simulink model "dcmotor_closedloop_inner_twoloop"  (R2022b)
settings: Solver=ode5  StartTime=0.0  StopTime=3  MaxStep=10e-6  RelTol=1e-1  EnableMultiTasking=on
libraries: spsDiodeLib x6, spsCurrentMeasurementLib x3, spsVoltageMeasurementLib x3, spsSeriesRLCBranchLib x3, spsACVoltageSourceLib x3, powerlib_extras x2, spsMosfetLib x2, spspowerguiLib x1, spsDCMachineLib x1, spsDCVoltageSourceLib x1, spsNeutralLib x1
settings Model: Creator=g0305973  LastModifiedBy=e0927009
settings SolverCC: AlgebraicLoopSolver=TrustRegion
settings DataIOCC: LimitDataPoints=on  SaveFormat=Array  SignalLoggingSaveFormat=ModelDataLogs  ReturnWorkspaceOutputs=off  SignalLoggingName=sigsOut
settings OptimizationCC: ExpressionDepthLimit=2147483647  InitFltsAndDblsToZero=on  LifeSpan=inf
settings DebuggingCC: SaveWithParameterizedLinksMsg=none  UnderspecifiedInitializationDetection=Classic  MergeDetectMultiDrivingBlocksExec=none  SignalResolutionControl=TryResolveAllWithWarning  MultiTaskDSMMsg=warning  MultiTaskCondExecSysMsg=none  FcnCallInpInsideContextMsg=warning  UnconnectedInputMsg=warning  UnconnectedOutputMsg=warning  UnconnectedLineMsg=warning  StateNameClashWarn=warning  SFUnexpectedBacktrackingDiag=warning  SFNoUnconditionalDefaultTransitionDiag=warning  SFExecutionAtInitializationDiag=none  SFMachineParentedDataDiag=warning  ArithmeticOperatorsInVariantConditions=warning
settings HardwareCC: ProdBitPerPointer=32  ProdBitPerSizeT=32  ProdBitPerPtrDiffT=32  ProdLargestAtomicFloat=None  ProdIntDivRoundTo=Undefined  ProdEndianess=Unspecified  ProdWordSize=32  ProdHWDeviceType=32-bit Generic  TargetUnknown=on
settings ModelReferenceCC: EnableRefExpFcnMdlSchedulingChecks=on  PropagateSignalLabelsOutOfModel=off
settings SFSimCC: SimUseLocalCustomCode=off  CustomCodeUndefinedFunction=UseInterfaceOnly
settings RTWCC: RTWUseLocalCustomCode=off
settings CodeAppCC: StateflowObjectComments=on
settings GRTTargetCC: TargetFcnLib=ansi_tfl_tmw.mat  TargetLangStandard=C89/C90 (ANSI)  CombineOutputUpdateFcns=off  GRTInterface=on
settings ConfigComp: CovMetricSettings=dw  CovSaveCumulativeToWorkspaceVar=on  CovSaveSingleToWorkspaceVar=on  CovExternalEMLEnable=off
settings SimscapeCC: SimscapeNormalizeSystem=off

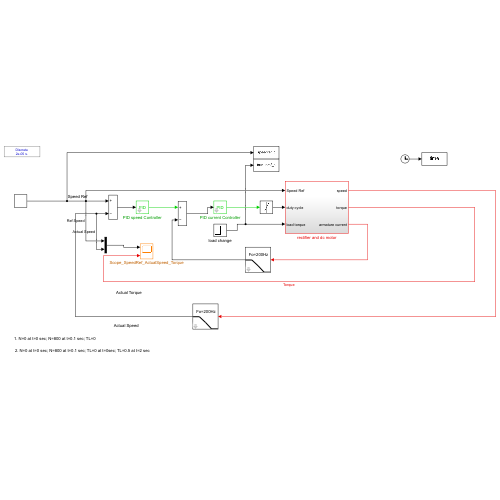
[thumbnail: Simulink's stored preview of the top-level diagram]
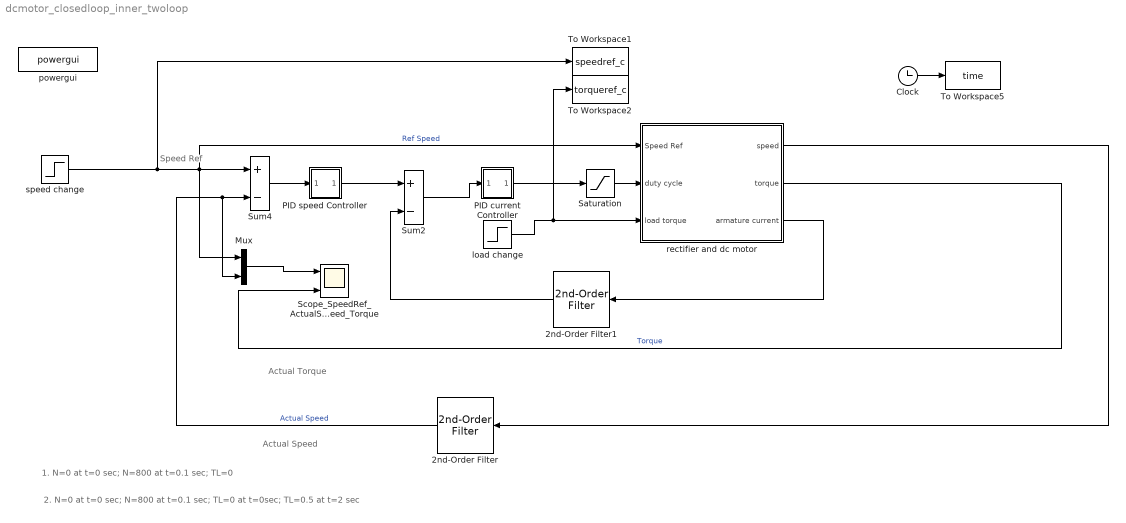
== system dcmotor_closedloop_inner_twoloop ==
  note: Speed Ref
  note: Actual Speed
  note: Actual Torque
  note: 2. N=0 at t=0 sec; N=800 at t=0.1 sec; TL=0 at t=0sec; TL=0.5 at t=2 sec
  note: 1. N=0 at t=0 sec; N=800 at t=0.1 sec; TL=0
  2nd-Order Filter : powerlib_extras/Control  Blocks/2nd-Order Filter  FilterType=Lowpass  Fo=200  Zeta=0.707  Initialize=off  Vac_Init=[1 45 60]  Vdc_Init=-0.5  PlotResponse=off  param1=[1 500 1]
  2nd-Order Filter1 : powerlib_extras/Control  Blocks/2nd-Order Filter  FilterType=Lowpass  Fo=200  Zeta=0.707  Initialize=off  Vac_Init=[1 45 60]  Vdc_Init=-0.5  PlotResponse=off  param1=[1 500 1]
  Clock : Clock
  Mux : Mux  Inputs=2
  PID current Controller : Subsystem  AncestorBlock=simulink_extras/Additional Linear/PID Controller  mask(PID Controller){P=0.4366, I=32.4627, D=0}
      mask prompts: P "Proportional:"; I "Integral:"; D "Derivative:"
      mask help:
      | Enter expressions for proportional, integral, and derivative terms.
      | P+I/s+Ds
      settings: LibrarySourceBlock=|
      | simulink_extras/Additional
      | Linear/PID Controller
      mask Help: This block implements a PID controller where parameters are entered for the Proportional, Integral and Derivative terms. Unmask this block to see how it works. The derivative term is implemented using a true derivative block.
      mask Display: disp('PID')
  PID speed Controller : Subsystem  AncestorBlock=simulink_extras/Additional Linear/PID Controller  mask(PID Controller){P=0.0256, I=0.0163, D=0}
      mask prompts: P "Proportional:"; I "Integral:"; D "Derivative:"
      mask help:
      | Enter expressions for proportional, integral, and derivative terms.
      | P+I/s+Ds
      settings: LibrarySourceBlock=|
      | simulink_extras/Additional
      | Linear/PID Controller
      mask Help: This block implements a PID controller where parameters are entered for the Proportional, Integral and Derivative terms. Unmask this block to see how it works. The derivative term is implemented using a true derivative block.
      mask Display: disp('PID')
  Saturation : Saturate  UpperLimit=1  LowerLimit=0
  Scope_SpeedRef_ActualSpeed_Torque : Scope  NumInputPorts=2
  Sum2 : Sum  Inputs=+-  SaturateOnIntegerOverflow=on
  Sum4 : Sum  Inputs=+-  SaturateOnIntegerOverflow=on
  To Workspace1 : ToWorkspace  VariableName=speedref_c  SampleTime=2e-5
  To Workspace2 : ToWorkspace  VariableName=torqueref_c  SampleTime=2e-5
  To Workspace5 : ToWorkspace  VariableName=time  SampleTime=2e-5
  load change : Step  Time=2  After=0.5  SampleTime=0
  powergui : spspowerguiLib/powergui  Priority=2  SimulationMode=Discrete  SampleTime=20e-6  frequency=60  Iterations=50  frequencyindice=50  Pbase=100e6  ErrMax=1e-4  UnitsV=kV  UnitsW=MW  buscounter=0  FunctionMessages=off  echomessages=off  EnableUseOfTLC=off  CurrentSourceSwitches=off  DisableSnubberDevices=off  DisableRonSwitches=off  DisableVfSwitches=off  DisplayEquations=off  AutomaticDiscreteSolvers=off  SolverType=Tustin  Interpol=off  ExternalGateDelay=off  methode=off  Ts=0  x0status=blocks  SPID=off  SwTol=0  HookPort=off  NonlinearTolerance=1e-4  nMaxIteration=100  ContinueOnMaxIteration=off  RestoreLinks=warning  ResistiveCurrentMeasurement=off  Frange=[0:2:500]  Ylog=off  Xlog=on  ShowGrid=off  save=off  variable=ZData  structure=0  ZoomFFT=on  StartTime=0.0  cycles=1  DisplayStyle=1  fundamental=60  FreqAxis=off  MaxFrequency=1000  frequencyindicesteady=1  RmsSteady=1  display=off
  rectifier and dc motor : Subsystem
  speed change : Step  Time=0.1  After=800  SampleTime=0
  wires:
  rectifier and dc motor/1(speed) -> 2nd-Order Filter/1
  Mux/1 -> Scope_SpeedRef_ActualSpeed_Torque/1
  Sum4/1 -> PID speed Controller/1(In_1)
  2nd-Order Filter/1 -> Sum4/2, Mux/2  "Actual Speed"
  speed change/1 -> Sum4/1, rectifier and dc motor/1(Speed Ref), Mux/1, To Workspace1/1  "Ref Speed"
  rectifier and dc motor/2(torque) -> Scope_SpeedRef_ActualSpeed_Torque/2  "Torque"
  load change/1 -> To Workspace2/1, rectifier and dc motor/3(load torque)
  Clock/1 -> To Workspace5/1
  Sum2/1 -> PID current Controller/1(In_1)
  rectifier and dc motor/3(armature current) -> 2nd-Order Filter1/1
  2nd-Order Filter1/1 -> Sum2/2
  PID current Controller/1(Out_1) -> Saturation/1
  PID speed Controller/1(Out_1) -> Sum2/1
  Saturation/1 -> rectifier and dc motor/2(duty cycle)

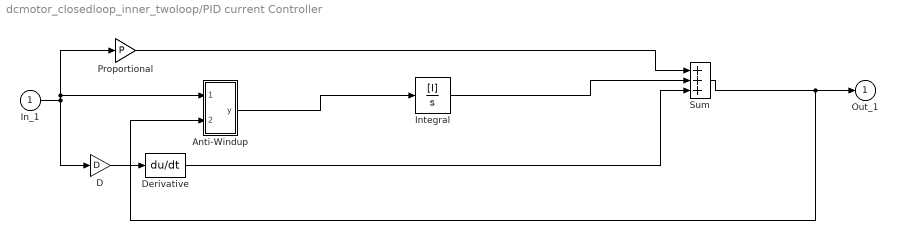
== system dcmotor_closedloop_inner_twoloop/PID current Controller ==
  In_1 : Inport
  Anti-Windup : Subsystem
  D : Gain  Gain=D  SaturateOnIntegerOverflow=on  OutDataTypeStr=Inherit: Same as input  ParamDataTypeStr=Inherit: Same as input
  Derivative : Derivative
  Integral : TransferFcn  Numerator=[I]  Denominator=[1 0]
  Proportional : Gain  Gain=P  SaturateOnIntegerOverflow=on  OutDataTypeStr=Inherit: Same as input  ParamDataTypeStr=Inherit: Same as input
  Sum : Sum  Inputs=+++  InputSameDT=on  SaturateOnIntegerOverflow=on  OutDataTypeStr=Inherit: Same as first input
  Out_1 : Outport  InitialOutput=0  VectorParamsAs1DForOutWhenUnconnected=off
  wires:
  Proportional/1 -> Sum/1
  Integral/1 -> Sum/2
  Derivative/1 -> Sum/3
  In_1/1 -> Anti-Windup/1(difference), Proportional/1, D/1
  Sum/1 -> Out_1/1, Anti-Windup/2(ctrl_out)
  D/1 -> Derivative/1
  Anti-Windup/1(y) -> Integral/1

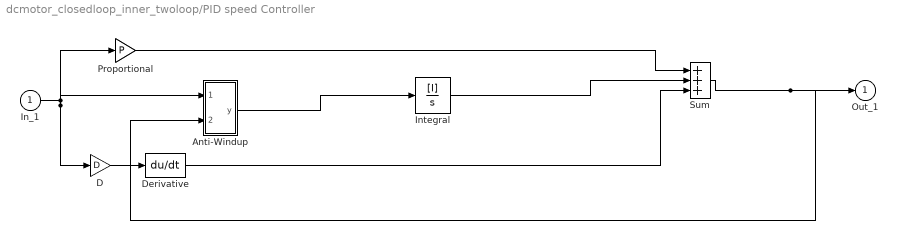
== system dcmotor_closedloop_inner_twoloop/PID speed Controller ==
  In_1 : Inport
  Anti-Windup : Subsystem
  D : Gain  Gain=D  SaturateOnIntegerOverflow=on  OutDataTypeStr=Inherit: Same as input  ParamDataTypeStr=Inherit: Same as input
  Derivative : Derivative
  Integral : TransferFcn  Numerator=[I]  Denominator=[1 0]
  Proportional : Gain  Gain=P  SaturateOnIntegerOverflow=on  OutDataTypeStr=Inherit: Same as input  ParamDataTypeStr=Inherit: Same as input
  Sum : Sum  Inputs=+++  InputSameDT=on  SaturateOnIntegerOverflow=on  OutDataTypeStr=Inherit: Same as first input
  Out_1 : Outport  InitialOutput=0  VectorParamsAs1DForOutWhenUnconnected=off
  wires:
  Proportional/1 -> Sum/1
  Integral/1 -> Sum/2
  Derivative/1 -> Sum/3
  In_1/1 -> Proportional/1, D/1, Anti-Windup/1(difference)
  Sum/1 -> Out_1/1, Anti-Windup/2(ctrl_out)
  D/1 -> Derivative/1
  Anti-Windup/1(y) -> Integral/1

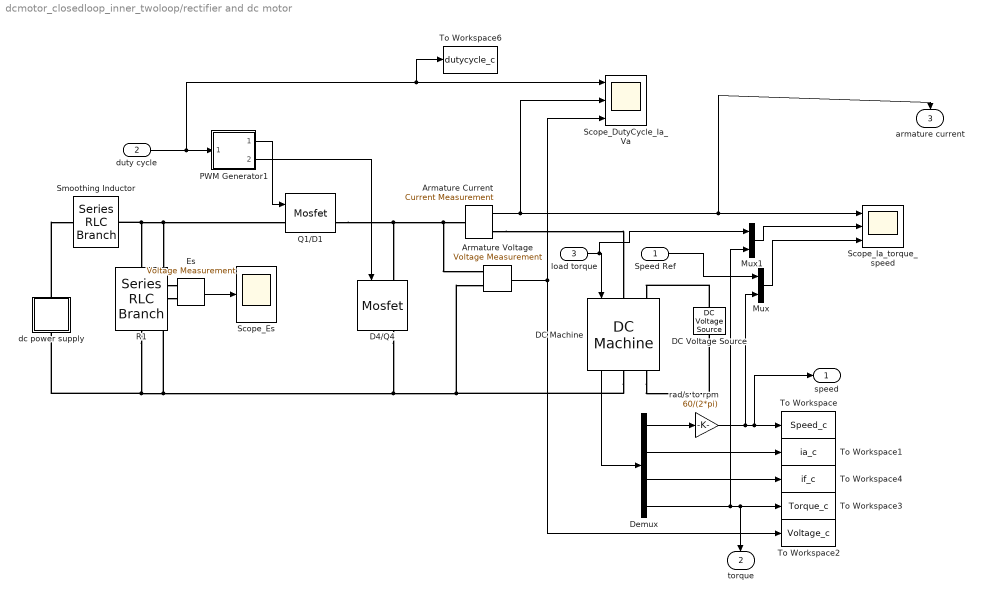
== system dcmotor_closedloop_inner_twoloop/rectifier and dc motor ==
  Speed Ref : Inport
  duty cycle : Inport  Port=2
  load torque : Inport  Port=3
  "Armature Current " : spsCurrentMeasurementLib/Current Measurement  Tag=PoWeRsYsTeMmEaSuReMeNt  PhasorSimulation=off  OutputType=Magnitude  PSBequivalent=0
      settings: AttributesFormatString=\n
  Armature Voltage : spsVoltageMeasurementLib/Voltage Measurement  Tag=PoWeRsYsTeMmEaSuReMeNt  PhasorSimulation=off  OutputType=Magnitude  PSBequivalent=0
  D4/Q4 : spsMosfetLib/Mosfet  Ron=0.001  Lon=0  Rd=0.01  Vfd=0  IC=0  Rs=10  Cs=inf  Measurements=on
  DC Machine : spsDCMachineLib/DC Machine  PresetModel=No  MechanicalLoad=Torque TL  FieldType=Wound  ShowDetailedParameters=on  MeasurementBus=off  RLa="[29  0.39]"  RLf="[697  14.9]"  Laf=1.8072  MachineConstant=Torque constant (N.m/A)  Ke=1.8  Kt=1.8  J=0.0024  Bm=0  Tf=0  w0=0  Ifinit=0.344332855093257  TsPowergui=0  TsBlock=-1
      settings: AttributesFormatString=\n
  DC Voltage Source : spsDCVoltageSourceLib/DC Voltage Source  Description=source block  Amplitude=240  Measurements=None
      settings: AttributesFormatString=\n
  Demux : Demux
      settings: DisplayOption=none
  Es : spsVoltageMeasurementLib/Voltage Measurement  Tag=PoWeRsYsTeMmEaSuReMeNt  PhasorSimulation=off  OutputType=Magnitude  PSBequivalent=0
  Mux : Mux  Inputs=2
  Mux1 : Mux  Inputs=2
  PWM Generator1 : Subsystem
      mask Display: plot([1,2,2,3,3,4,4,5,5,6],[0,0,5,5,0,0,5,5,0,0])
  Q1/D1 : spsMosfetLib/Mosfet  Ron=0.001  Lon=0  Rd=0.01  Vfd=0  IC=0  Rs=10  Cs=inf  Measurements=on
  R1 : spsSeriesRLCBranchLib/Series RLC Branch  LConnTagsString=__new0  RConnTagsString=__new0  BranchType=R  Resistance=455e10  Inductance=1.0  SetiL0=off  InitialCurrent=0  Capacitance=1.0  Setx0=off  InitialVoltage=0  Measurements=None
  Scope_DutyCycle_Ia_Va : Scope  NumInputPorts=3
  Scope_Es : Scope
  Scope_Ia_torque_speed : Scope  NumInputPorts=3
  Smoothing Inductor : spsSeriesRLCBranchLib/Series RLC Branch  LConnTagsString=__new0  RConnTagsString=__new0  BranchType=L  Resistance=1.0  Inductance=0.8  SetiL0=off  InitialCurrent=0  Capacitance=1.0  Setx0=off  InitialVoltage=0  Measurements=Branch voltage
  To Workspace : ToWorkspace  VariableName=Speed_c  SampleTime=2e-5
  To Workspace1 : ToWorkspace  VariableName=ia_c  SampleTime=2e-5
  To Workspace2 : ToWorkspace  VariableName=Voltage_c  SampleTime=2e-5
  To Workspace3 : ToWorkspace  VariableName=Torque_c  SampleTime=2e-5
  To Workspace4 : ToWorkspace  VariableName=if_c  SampleTime=2e-5
  To Workspace6 : ToWorkspace  VariableName=dutycycle_c  SampleTime=2e-5
  dc power supply : Subsystem
  rad/s to rpm : Gain  Gain=60/(2*pi)  SaturateOnIntegerOverflow=on  OutDataTypeStr=Inherit: Same as input  ParamDataTypeStr=Inherit: Same as input
  speed : Outport  VectorParamsAs1DForOutWhenUnconnected=off
  torque : Outport  Port=2  VectorParamsAs1DForOutWhenUnconnected=off
  armature current : Outport  Port=3  VectorParamsAs1DForOutWhenUnconnected=off
  wires:
  duty cycle/1 -> PWM Generator1/1(DutyCycle), Scope_DutyCycle_Ia_Va/1, To Workspace6/1
  Demux/1 -> rad/s to rpm/1
  Demux/4 -> To Workspace3/1, torque/1, Mux1/2
  PWM Generator1/1(Gate pulse top switch) -> Q1/D1/1
  PWM Generator1/2(Gate pulse bottom switch) -> D4/Q4/1
  Demux/2 -> To Workspace1/1
  Demux/3 -> To Workspace4/1
  DC Machine/1 -> Demux/1
  Armature Voltage/1 -> To Workspace2/1, Scope_DutyCycle_Ia_Va/3
  Es/1 -> Scope_Es/1
  load torque/1 -> Mux1/1, DC Machine/1
  "Armature Current "/1 -> Scope_DutyCycle_Ia_Va/2, Scope_Ia_torque_speed/1, armature current/1
  Mux/1 -> Scope_Ia_torque_speed/3
  rad/s to rpm/1 -> Mux/2, To Workspace/1, speed/1
  Speed Ref/1 -> Mux/1
  Mux1/1 -> Scope_Ia_torque_speed/2
  connections:
  Es/LConn2 -- R1/RConn1 -- dc power supply/RConn1 -- DC Machine/RConn1 -- Armature Voltage/LConn2 -- D4/Q4/RConn1
  Es/LConn1 -- R1/LConn1 -- Smoothing Inductor/RConn1 -- Q1/D1/LConn1
  D4/Q4/LConn1 -- Q1/D1/RConn1 -- "Armature Current "/LConn1 -- Armature Voltage/LConn1
  DC Voltage Source/RConn1 -- DC Machine/LConn2
  "Armature Current "/RConn1 -- DC Machine/LConn1
  DC Machine/RConn2 -- DC Voltage Source/LConn1
  dc power supply/LConn1 -- Smoothing Inductor/LConn1

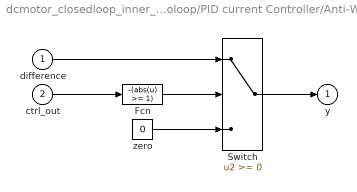
== system dcmotor_closedloop_inner_twoloop/PID current Controller/Anti-Windup ==
  difference : Inport
  ctrl_out : Inport  Port=2
  Fcn : Fcn  Expr=-(abs(u) >= 1)
  Switch : Switch
  zero : Constant  Value=0
  y : Outport  VectorParamsAs1DForOutWhenUnconnected=off
  wires:
  zero/1 -> Switch/3
  Fcn/1 -> Switch/2
  ctrl_out/1 -> Fcn/1
  difference/1 -> Switch/1
  Switch/1 -> y/1

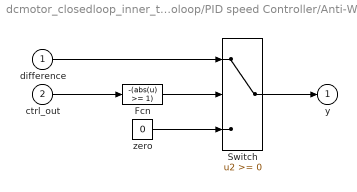
== system dcmotor_closedloop_inner_twoloop/PID speed Controller/Anti-Windup ==
  difference : Inport
  ctrl_out : Inport  Port=2
  Fcn : Fcn  Expr=-(abs(u) >= 1)
  Switch : Switch
  zero : Constant  Value=0
  y : Outport  VectorParamsAs1DForOutWhenUnconnected=off
  wires:
  zero/1 -> Switch/3
  Fcn/1 -> Switch/2
  ctrl_out/1 -> Fcn/1
  difference/1 -> Switch/1
  Switch/1 -> y/1

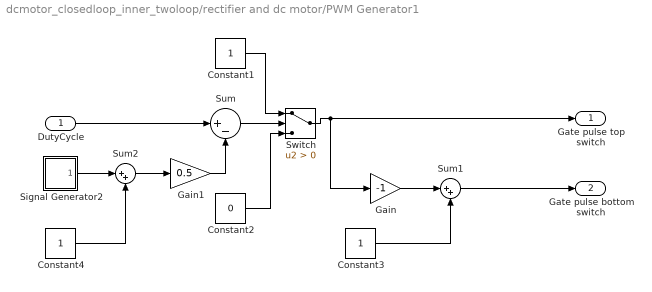
== system dcmotor_closedloop_inner_twoloop/rectifier and dc motor/PWM Generator1 ==
  DutyCycle : Inport
  Constant1 : Constant
  Constant2 : Constant  Value=0
  Constant3 : Constant
  Constant4 : Constant
  Gain : Gain  Gain=-1  SaturateOnIntegerOverflow=on  OutDataTypeStr=Inherit: Same as input  ParamDataTypeStr=Inherit: Same as input
  Gain1 : Gain  Gain=0.5  SaturateOnIntegerOverflow=on  OutDataTypeStr=Inherit: Same as input  ParamDataTypeStr=Inherit: Same as input
  Signal Generator2 : Subsystem  mask(DiscretizedSignalGenerator){WaveForm=sawtooth, Amplitude=1, Frequency=2000, Units=Hertz, SampleTime=20e-6}
      mask prompts: SampleTime "Sample time:"
      mask help: A discrete equivalent to the Signal Generator Block.
      mask init:
      | xdrw = 11*[1,1,2,2,1];
      | ydrw = [72,88,88,72,72];
      | xcirc = 11*[0,0,0.25,0.75,1,1,0.75,0.25,0];
      | ycirc = 16*[0.25,0.75,1,1,0.75,0.25,0,0,0.25];
      | switch Units
      |   case 'rad/sec'
      |     frequencyHz = Frequency/(2*pi);
      |     frequencyRads = Frequency;
      |   case 'Hertz'
      |     frequencyHz = Frequency;
      |     frequencyRads = Frequency*2*pi;
      | end
      | Period = 1.0/frequencyHz;
      | st=SampleTime;
      | DupSampleTime = SampleTime;
      | if length(SampleTime) > 1
      |     st=SampleTime(1);
      | end
      | %discretePeriod = round(period/st);
      | %pulseWidth = round(period*duty/100/st);
      | %phaseDelay =round(start/st);
      | %SampleTime=st;
      | if(st > 0)
      |     PeriodSamples = max(2,round(Period/st));
      |     halfSamples = max(1,round(PeriodSamples/2));
      | else
      | 	PeriodSamples = 2;
      |     halfSamples = 1;
      | end
      | 
      | sldiscutil('initsiggenmask', st);
      mask TypeOptions WaveForm: sine | square | sawtooth | random
      mask TypeOptions Units: rad/sec | Hertz
      mask Display:
      | plot( 1,1,99,99,   0+xdrw, ydrw );
      | plot( 1,1,99,99, 22+xdrw, ydrw );
      | plot( 1,1,99,99, 44+xdrw, ydrw );
      | plot( 1,1,99,99, 66+xdrw, ydrw );
      | plot( 1,1,99,99, 22+xcirc, 44+ycirc );
      | plot( 1,1,99,99, 44+xcirc, 44+ycirc );
  Sum : Sum  Inputs=|+-  SaturateOnIntegerOverflow=on
  Sum1 : Sum  Inputs=|++  SaturateOnIntegerOverflow=on
  Sum2 : Sum  Inputs=|++  SaturateOnIntegerOverflow=on
  Switch : Switch  Criteria=u2 > Threshold  InputSameDT=off
  Gate pulse top switch : Outport  VectorParamsAs1DForOutWhenUnconnected=off
  Gate pulse bottom switch : Outport  Port=2  VectorParamsAs1DForOutWhenUnconnected=off
  wires:
  Constant3/1 -> Sum1/2
  Gain/1 -> Sum1/1
  Switch/1 -> Gate pulse top switch/1, Gain/1
  Constant2/1 -> Switch/3
  Constant1/1 -> Switch/1
  Sum/1 -> Switch/2
  Sum1/1 -> Gate pulse bottom switch/1
  Signal Generator2/1(Out1) -> Sum2/1
  Constant4/1 -> Sum2/2
  Sum2/1 -> Gain1/1
  DutyCycle/1 -> Sum/1
  Gain1/1 -> Sum/2

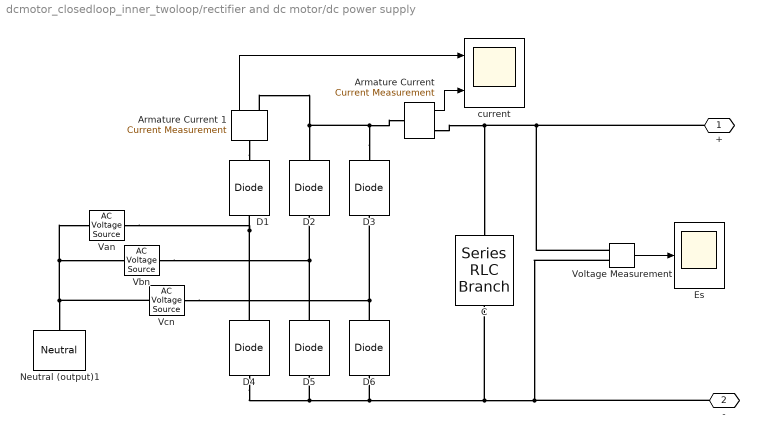
== system dcmotor_closedloop_inner_twoloop/rectifier and dc motor/dc power supply ==
  "Armature Current " : spsCurrentMeasurementLib/Current Measurement  Tag=PoWeRsYsTeMmEaSuReMeNt  PhasorSimulation=off  OutputType=Magnitude  PSBequivalent=0
      settings: AttributesFormatString=\n
  Armature Current 1 : spsCurrentMeasurementLib/Current Measurement  Tag=PoWeRsYsTeMmEaSuReMeNt  PhasorSimulation=off  OutputType=Magnitude  PSBequivalent=0
      settings: AttributesFormatString=\n
  C : spsSeriesRLCBranchLib/Series RLC Branch  LConnTagsString=__new0  RConnTagsString=__new0  BranchType=C  Resistance=1.0  Inductance=1.0  SetiL0=off  InitialCurrent=0  Capacitance=10000e-6  Setx0=off  InitialVoltage=0  Measurements=None
  D{1..6} (6 alike) : spsDiodeLib/Diode  Ron=1e-3  Lon=0  Vf=0.8  IC=0  UseSnubber=off  Rs=1e5  Cs=inf  Measurements=off
  Es : Scope
  Neutral (output)1 : spsNeutralLib/Neutral  LConnTagsString=a  NodeNumber=99
      settings: AttributesFormatString=node %<NodeNumber>  LibrarySourceBlock=sps_lib/Utilities/Neutral
  Van : spsACVoltageSourceLib/AC Voltage Source  Description=source block  Amplitude=240*1.414  Phase=0  Frequency=50  SampleTime=0  Measurements=None  BusType=swing  Pref=10e3  Qref=0  Qmin=-inf  Qmax=+inf
      settings: AttributesFormatString=\n
  Vbn : spsACVoltageSourceLib/AC Voltage Source  Description=source block  Amplitude=240*1.414  Phase=-120  Frequency=50  SampleTime=0  Measurements=None  BusType=swing  Pref=10e3  Qref=0  Qmin=-inf  Qmax=+inf
      settings: AttributesFormatString=\n
  Vcn : spsACVoltageSourceLib/AC Voltage Source  Description=source block  Amplitude=240*1.414  Phase=120  Frequency=50  SampleTime=0  Measurements=None  BusType=swing  Pref=10e3  Qref=0  Qmin=-inf  Qmax=+inf
      settings: AttributesFormatString=\n
  Voltage Measurement : spsVoltageMeasurementLib/Voltage Measurement  PhasorSimulation=off  OutputType=Complex  PSBequivalent=0
  current : Scope  NumInputPorts=2
  + : PMIOPort  Side=Left
  - : PMIOPort  Port=2  Side=Right
  wires:
  Voltage Measurement/1 -> Es/1
  Armature Current 1/1 -> current/1
  "Armature Current "/1 -> current/2
  connections:
  D3/RConn1 -- "Armature Current "/LConn1 -- D2/RConn1 -- Armature Current 1/RConn1
  D4/RConn1 -- Van/RConn1 -- D1/LConn1
  D5/RConn1 -- D2/LConn1 -- Vbn/RConn1
  D6/RConn1 -- D3/LConn1 -- Vcn/RConn1
  C/RConn1 -- Voltage Measurement/LConn2 -- -/RConn1 -- D6/LConn1 -- D4/LConn1 -- D5/LConn1
  Vcn/LConn1 -- Van/LConn1 -- Vbn/LConn1 -- Neutral (output)1/LConn1
  +/RConn1 -- "Armature Current "/RConn1 -- C/LConn1 -- Voltage Measurement/LConn1
  Armature Current 1/LConn1 -- D1/RConn1

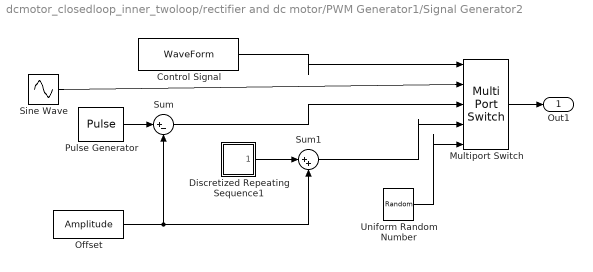
== system dcmotor_closedloop_inner_twoloop/rectifier and dc motor/PWM Generator1/Signal Generator2 ==
  Control Signal : Constant  Value=WaveForm
  Discretized Repeating Sequence1 : Subsystem  AncestorBlock=discretizing/Discretized Repeating Sequence  mask(DiscretizedRepeatingTable){rep_seq_t=[0 Period], rep_seq_y=[0 ((-2)*Amplitude)], SampleTime=DupSampleTime}
      mask prompts: rep_seq_t "Time values:"; rep_seq_y "Output values:"; SampleTime "Sample time:"
      mask help: Repeating table.
      mask init:
      | period = max(rep_seq_t);
      | st=SampleTime;
      | if length(st)>1
      |     st=SampleTime(1);
      | end
      | sldiscutil('initrepeatsequencemask', st);
      settings: LibrarySourceBlock=|
      | discretizing/Discretized
      | Repeating Sequence
      mask Help: Repeats cycle given in table. Time values should be monotonically increasing.
      mask Display: plot([rep_seq_t,rep_seq_t+period,rep_seq_t+2*period,rep_seq_t(1)+3*period],[rep_seq_y,rep_seq_y,rep_seq_y,rep_seq_y(1)])
  Multiport Switch : MultiPortSwitch  Inputs=4  SaturateOnIntegerOverflow=off
  Offset : Constant  Value=Amplitude
  Pulse Generator : DiscretePulseGenerator  Amplitude=2*Amplitude  Period=PeriodSamples  PulseWidth=halfSamples  PhaseDelay=halfSamples  SampleTime=st
  Sine Wave : Sin  Amplitude=Amplitude  Frequency=frequencyRads  SampleTime=SampleTime
  Sum : Sum  Inputs=|+-  InputSameDT=on  SaturateOnIntegerOverflow=on  OutDataTypeStr=Inherit: Same as first input
  Sum1 : Sum  Inputs=|++  InputSameDT=on  SaturateOnIntegerOverflow=on  OutDataTypeStr=Inherit: Same as first input
  Uniform Random Number : UniformRandomNumber  Minimum=(-1)*Amplitude  Maximum=Amplitude  SampleTime=SampleTime
  Out1 : Outport  VectorParamsAs1DForOutWhenUnconnected=off
  wires:
  Offset/1 -> Sum/2, Sum1/2
  Sum1/1 -> Multiport Switch/4
  Discretized Repeating Sequence1/1(Out1) -> Sum1/1
  Multiport Switch/1 -> Out1/1
  Sum/1 -> Multiport Switch/3
  Pulse Generator/1 -> Sum/1
  Control Signal/1 -> Multiport Switch/1
  Sine Wave/1 -> Multiport Switch/2
  Uniform Random Number/1 -> Multiport Switch/5

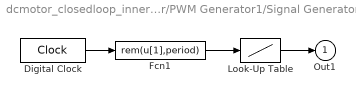
== system dcmotor_closedloop_inner_twoloop/rectifier and dc motor/PWM Generator1/Signal Generator2/Discretized Repeating Sequence1 ==
  Digital Clock : DigitalClock  SampleTime=SampleTime
  Fcn1 : Fcn  Expr=rem(u[1],period)
  Look-Up Table : Lookup  InputValues=rep_seq_t  Table=rep_seq_y
  Out1 : Outport  VectorParamsAs1DForOutWhenUnconnected=off
  wires:
  Look-Up Table/1 -> Out1/1
  Digital Clock/1 -> Fcn1/1
  Fcn1/1 -> Look-Up Table/1
